simulink model "blockDiagramTask3"  (R2025a)
settings: Solver=VariableStepAuto  StartTime=0.0  StopTime=0.001  RelTol=1e-3
InitFcn:
  | run motor_specs.m
model workspace: external: MATLAB File motor_specs.m (data not in the file)
values from neighbouring files (symbols this model uses):
  A = [(-R/L), (-K_E/L); K_M/J, (-b_m/J)]    [motor_specs.m]    (also in ssAndTF.m = -((K_M*K_E + (C_V*R))/(J*R)))
  B = [(1/L), 0]'    [motor_specs.m]    (also in ssAndTF.m = K_M/ (J * R))
  b_m = C_V / rpm_to_rs    (= 1.05042262441e-05)    [motor_specs.m]
  C = [0, 1]    [motor_specs.m]    (also in ssAndTF.m = 1)
  D = 0    [motor_specs.m]    (also in ssAndTF.m)
  J = 6.3E-6    (= 6.3e-06)    [motor_specs.m]
  K_E = 0.006741 / rpm_to_rs    (= 0.0643718082829)    [motor_specs.m]
  K_M = 0.0644    [motor_specs.m]
  L = 0.000238    [motor_specs.m]
  R = 3.23    [motor_specs.m]
libraries: fl_lib x4, nesl_utility x3, ee_lib x1
settings Model: Creator=josef  LastModifiedBy=josef

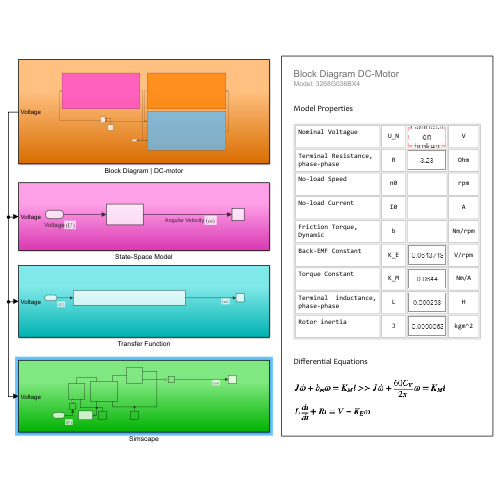
[thumbnail: Simulink's stored preview of the top-level diagram]
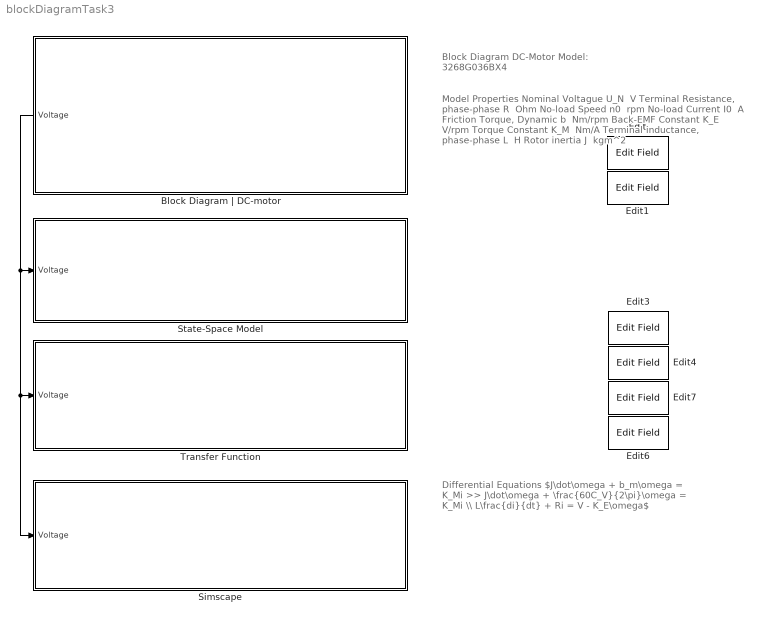
== system blockDiagramTask3 ==
  note: Differential Equations
      |
      | $J\dot\omega + b_m\omega = K_Mi >> J\dot\omega + \frac{60C_V}{2\pi}\omega = K_Mi \\ L\frac{di}{dt} + Ri = V - K_E\omega$
  note: Model Properties
      |
      | Nominal Voltague
      |
      | U_N
      | ​
      | V
      |
      | Terminal Resistance,
      | phase-phase
      | R
      | ​
      | Ohm
      |
      | No-load Speed
      |
      | n0
      | ​
      | rpm
      |
      | No-load Current
      |
      | I0
      | ​
      | A
      |
      | Friction Torque,
      | Dynamic
      | b
      | ​
      | Nm/rpm
      |
      | Back-EMF Constant
      |
      | K_E
      | ​
      | V/rpm
      |
      | Torque Constant
      |
      | K_M
      | ​
      | Nm/A
      |
      | Terminal inductance,
      | phase-phase
      | L
      | ​
      | H
      |
      | Rotor inertia
      |
      | J
      | ​
      | kgm^2
  note: Block Diagram DC-Motor
      | Model: 3268G036BX4
  Block Diagram | DC-motor : Subsystem
      settings: PortSchema="{\"entries\":[{\"content\":{\"sides\":[{\"content\":{\"connectorIds\":[\"Out1\"]},\"type\":\"ConnectorPlacement.EquallySpacedRectSide\",\"uuid\":\"f5369081-1a9d-45ec-910c-203cc00c981f\"},{\"content\":{\"side\":\"RIGHT\"},\"type\":\"ConnectorPlacement.EquallySpacedRectSide\",\"uuid\":\"7a9e2678-a5f9-47e4-b1dd-3d246fe1e19e\"},{\"content\":{\"side\":\"TOP\"},\"type\":\"ConnectorPlacement.EquallySpacedRectSide\",\"uuid\":\"9df29022-cccd-4d0c-afa1-a82374d6f5d8\"}]},\"type\":\"ConnectorPlacement.EquallySpacedConnector\",\"uuid\":\"5e82b34e-0277-45d8-be44-5ce71af6e010\"}],\"packageUris\":[\"http://schema.mathworks.com/mf0/Connector/R2020b\"],\"version\":\"1.0\"}"
  Edit{,1,3..4,6..7} (6 alike) : EditField  LabelPosition=Hide  ShowInitialText=on  Alignment=Center  Opacity=0
  Simscape : Subsystem
  State-Space Model : Subsystem
  Transfer Function : Subsystem
  wires:
  Block Diagram | DC-motor/1(Voltage) -> Simscape/1(Voltage), Transfer Function/1(Voltage), State-Space Model/1(Voltage)

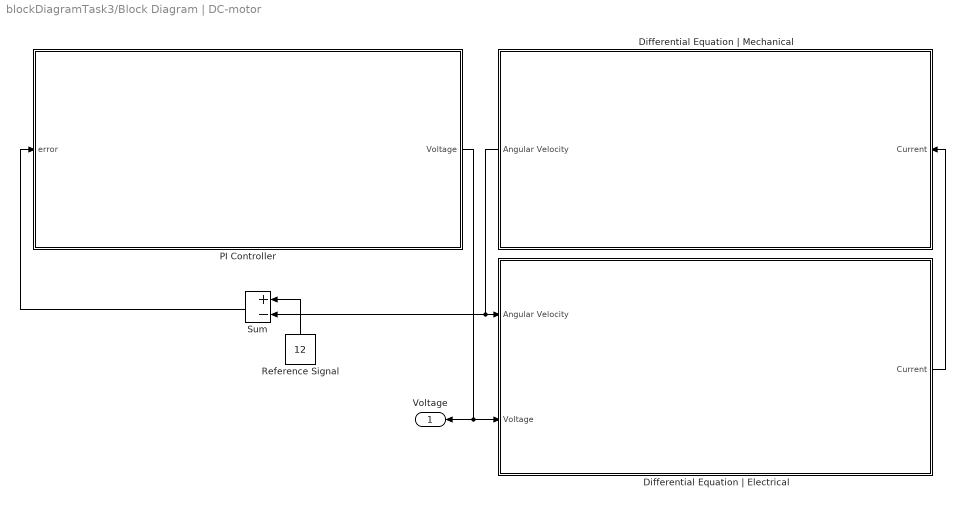
== system blockDiagramTask3/Block Diagram | DC-motor ==
  Differential Equation | Electrical : Subsystem
  Differential Equation | Mechanical : Subsystem
  PI Controller : Subsystem
  Reference Signal : Constant  Value=12
  Sum : Sum  Inputs=+-
  Voltage : Outport
  wires:
  Differential Equation | Electrical/1(Current) -> Differential Equation | Mechanical/1(Current)
  Reference Signal/1 -> Sum/1
  Differential Equation | Mechanical/1(Angular Velocity) -> Differential Equation | Electrical/1(Angular Velocity), Sum/2
  Sum/1 -> PI Controller/1(error)
  PI Controller/1(Voltage) -> Voltage/1, Differential Equation | Electrical/2(Voltage)

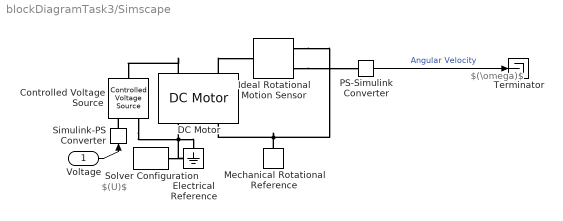
== system blockDiagramTask3/Simscape ==
  note: $(\omega)$
  note: $(U)$
  Voltage : Inport
  Controlled Voltage Source : fl_lib/Electrical/Electrical Sources/Controlled Voltage Source
  DC Motor : ee_lib/Electromechanical/Brushed Motors/DC Motor  field_option=ee.enum.field_option.pm  Rf=100 Ohm  Lf=1 H  Laf=0.15 H  If0=0 A  parameterization=ee.enum.dcparam_option.circuit_param  Ra=R Ohm  La=L H  emf_or_torque=ee.enum.emf_or_torque.kv  Kv=K_E V*s/rad  Ki=6.876e-4 N*m/A  T_stall=0.24e-3 N*m  w_max=19100 rpm  w_rated=15000 rpm  P_rated=0.08 W  V_rated=1.5 V  lam_param=ee.enum.lam_param.damping  i_noload=0 A  V_i_noload=1.5 V  J=J kg*m^2  lam=b_m N*m*s/rad  speed0=0 rpm  alpha=3.93e-3 1/K  Tmeas=25 degC  thermal_mass=100 J/K  initial_temperature=25 degC
  Electrical Reference : fl_lib/Electrical/Electrical Elements/Electrical Reference
  Ideal Rotational Motion Sensor : fl_lib/Mechanical/Mechanical Sensors/Ideal Rotational Motion Sensor  reference=foundation.enum.MeasurementReference.difference  acceleration_port=false  velocity_port=true  position_port=false  wrap_angle=false  offset=0 rad
      settings: InternalSimscapePortConfiguration="{\"Bottom\":[],\"Left\":[{\"id\":\"R\",\"label\":\"R\",\"type\":\"foundation.mechanical.rotational.rotational\"}],\"Right\":[{\"id\":\"C\",\"label\":\"C\",\"type\":\"foundation.mechanical.rotational.rotational\"},{\"id\":\"W\",\"label\":\"W\",\"type\":\"output\"}],\"Top\":[]}"
  Mechanical Rotational Reference : fl_lib/Mechanical/Rotational Elements/Mechanical Rotational Reference
  PS-Simulink Converter : nesl_utility/PS-Simulink Converter  PhysicalDomain=network_engine_domain  SubClassName=ps_output  LeftPortType=input  RightPortType=output  PseudoPeriodic=off  Frequencies=[]  VectorFormat=inherit  Unit=inherit  AffineConversion=off
  Simulink-PS Converter : nesl_utility/Simulink-PS Converter  PhysicalDomain=network_engine_domain  SubClassName=ps_input  LeftPortType=input  RightPortType=output  PseudoPeriodic=off  Frequencies=[]  NoiseDistribution=none  NoiseParameters=[]  Unit=1  AffineConversion=off  FilteringAndDerivatives=provide  SimscapeFilterOrder=1  InputFilterTimeConstant=0.001  UdotUserProvided=0
  Solver Configuration : nesl_utility/Solver Configuration  PhysicalDomain=network_engine_domain  SubClassName=solver  LeftPortType=input  RightPortType=generic  Tones=[]  Harmonics=[]  SimulateNoise=off  Profile=off  UseLocalSampling=off  EnableSwitchedLinearOptims=on  FrequencyDomain=off  UseCCode=off  RelTol=0.001  AbsTol=0.001  MinStep=1e-09  ToWorkspace=off  RevertToSquareIcSolve=off  NumHomotopyIterations=100  PhasorMode=off  PhasorModeNumHarmonics=1  ConsistencySolver=NEWTON_XTOL_AFTER_FTOL  IndexReductionMethod=DerivativeReplacement  DoDC=off  ResidualTolerance=1e-09  ConsistencyTolSource=GLOBAL  ConsistencyAbsTol=0.001  ConsistencyRelTol=0.001  ConsistencyTolFactor=0.001  UseLocalSolver=off  LocalSolverChoice=NE_BACKWARD_EULER_ADVANCER  ResolveIndetEquations=on  FunctionEvalNumThread=1  LocalSolverSampleTime=0.001  DoFixedCost=off  MaxNonlinIter=3  MaxModeIter=2  ComputeImpulses=off  ImpulseIterations=2  LinearAlgebra=auto  LinearAlgebraNumThread=0  EquationFormulation=NE_TIME_EF  DelaysMemoryBudget=1024  AutomaticFiltering=on  FilteringTimeConstant=0.001  PartitionStorageMethod=AS_NEEDED  PartitionMemoryBudget=1024  PartitionMethod=ROBUST  MultibodyUseLocalSolver=off  MultibodyLocalSolverChoice=ODE1  MultibodyLocalSolverSampleTime=0.001
  Terminator : Terminator
  wires:
  Voltage/1 -> Simulink-PS Converter/1
  PS-Simulink Converter/1 -> Terminator/1  "Angular Velocity"
  connections:
  Mechanical Rotational Reference/LConn1 -- Ideal Rotational Motion Sensor/RConn1 -- DC Motor/RConn2
  Solver Configuration/RConn1 -- Controlled Voltage Source/RConn2 -- Electrical Reference/LConn1 -- DC Motor/RConn1
  DC Motor/LConn2 -- Ideal Rotational Motion Sensor/LConn1
  DC Motor/LConn1 -- Controlled Voltage Source/LConn1
  Simulink-PS Converter/RConn1 -- Controlled Voltage Source/RConn1
  Ideal Rotational Motion Sensor/RConn2 -- PS-Simulink Converter/LConn1

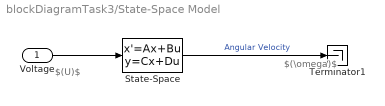
== system blockDiagramTask3/State-Space Model ==
  note: $(\omega)$
  note: $(U)$
  Voltage : Inport
  State-Space : StateSpace  A=A  B=B  C=C  D=D  InitialCondition=0
  Terminator1 : Terminator
  wires:
  State-Space/1 -> Terminator1/1  "Angular Velocity"
  Voltage/1 -> State-Space/1

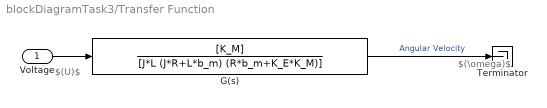
== system blockDiagramTask3/Transfer Function ==
  note: $(\omega)$
  note: $(U)$
  Voltage : Inport
  G(s) : TransferFcn  Numerator=[K_M]  Denominator=[J*L (J*R+L*b_m) (R*b_m+K_E*K_M)]
  Terminator : Terminator
  wires:
  G(s)/1 -> Terminator/1  "Angular Velocity"
  Voltage/1 -> G(s)/1

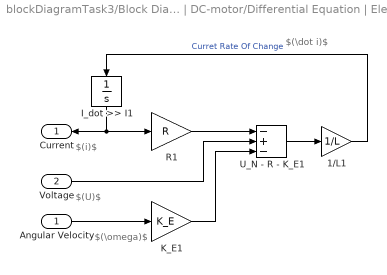
== system blockDiagramTask3/Block Diagram | DC-motor/Differential Equation | Electrical ==
  note: $(U)$
  note: $(i)$
  note: $(\dot i)$
  note: $(\omega)$
  Angular Velocity : Inport
  Voltage : Inport  Port=2
  1/L1 : Gain  Gain=1/L
  I_dot >> I1 : Integrator
  K_E1 : Gain  Gain=K_E
  R1 : Gain  Gain=R
  U_N - R - K_E1 : Sum  Inputs=-+-
  Current : Outport
  wires:
  1/L1/1 -> I_dot >> I1/1  "Curret Rate Of Change"
  U_N - R - K_E1/1 -> 1/L1/1
  K_E1/1 -> U_N - R - K_E1/3
  Angular Velocity/1 -> K_E1/1
  R1/1 -> U_N - R - K_E1/1
  I_dot >> I1/1 -> R1/1, Current/1
  Voltage/1 -> U_N - R - K_E1/2

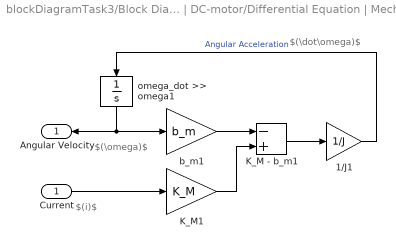
== system blockDiagramTask3/Block Diagram | DC-motor/Differential Equation | Mechanical ==
  note: $(\omega)$
  note: $(\dot\omega)$
  note: $(i)$
  Current : Inport
  1/J1 : Gain  Gain=1/J
  K_M - b_m1 : Sum  Inputs=-+
  K_M1 : Gain  Gain=K_M
  b_m1 : Gain  Gain=b_m
  omega_dot >> omega1 : Integrator
  Angular Velocity : Outport
  wires:
  K_M1/1 -> K_M - b_m1/2
  1/J1/1 -> omega_dot >> omega1/1  "Angular Acceleration"
  b_m1/1 -> K_M - b_m1/1
  K_M - b_m1/1 -> 1/J1/1
  Current/1 -> K_M1/1
  omega_dot >> omega1/1 -> b_m1/1, Angular Velocity/1

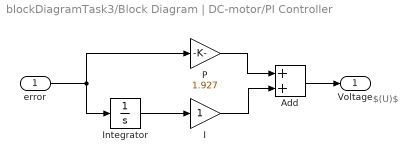
== system blockDiagramTask3/Block Diagram | DC-motor/PI Controller ==
  note: $(U)$
  error : Inport
  Add : Sum
  I : Gain
  Integrator : Integrator
  P : Gain  Gain=1.927
  Voltage : Outport
  wires:
  error/1 -> Integrator/1, P/1
  P/1 -> Add/1
  I/1 -> Add/2
  Add/1 -> Voltage/1
  Integrator/1 -> I/1
